simulink model "emldemo_led_switch"  (R2015a)
settings: Solver=FixedStepDiscrete  StartTime=0.0  StopTime=9  FixedStep=1  RelTol=1e-3
settings Model: CovSFcnEnable=off  Creator=The MathWorks, Inc.  LastModifiedBy=ktrinh
settings OptimizationCC: ExpressionDepthLimit=2147483647
settings DebuggingCC: UnderspecifiedInitializationDetection=Classic  MergeDetectMultiDrivingBlocksExec=none  SolverPrmCheckMsg=warning  FcnCallInpInsideContextMsg=EnableAllAsWarning  StateNameClashWarn=warning  StrictBusMsg=Warning
settings SFSimCC: SimParseCustomCode=off
settings GRTTargetCC: CombineOutputUpdateFcns=off  GRTInterface=on

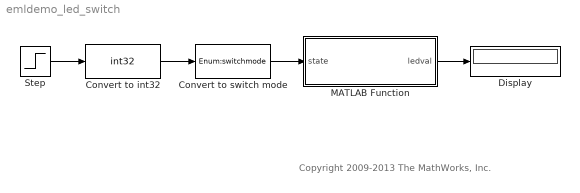
== system emldemo_led_switch ==
  note: Copyright 2009-2013 The MathWorks, Inc.
  Convert to int32 : DataTypeConversion  OutMin=0  OutMax=1  OutDataTypeStr=int32
  Convert to switch mode : DataTypeConversion  OutDataTypeStr=Enum:switchmode  SaturateOnIntegerOverflow=on
  Display : Display
  MATLAB Function : MATLAB Function  TreatAsAtomicUnit=on
      settings: PermitHierarchicalResolution=ParametersOnly
  Step : Step  SampleTime=10
  wires:
  MATLAB Function/1(ledval) -> Display/1
  Convert to switch mode/1 -> MATLAB Function/1(state)
  Step/1 -> Convert to int32/1
  Convert to int32/1 -> Convert to switch mode/1

== matlab function emldemo_led_switch/MATLAB Function ==
  data: state input; ledval output Enum: led
function ledval = checkState(state)
%#codegen

if state == switchmode.ON
    ledval = led.GREEN;
else
    ledval = led.RED;
end
